simulink model "massdamper"  (R2023a)
settings: Solver=VariableStepAuto  StartTime=0.0  StopTime=10.0  RelTol=1e-3
values from neighbouring files (symbols this model uses):
  k = 1    [RCTF.m]
undefined symbols (not defined in the file or in its folder): b, m
settings Model: Creator=Egypt_Laptop  LastModifiedBy=Egypt_Laptop

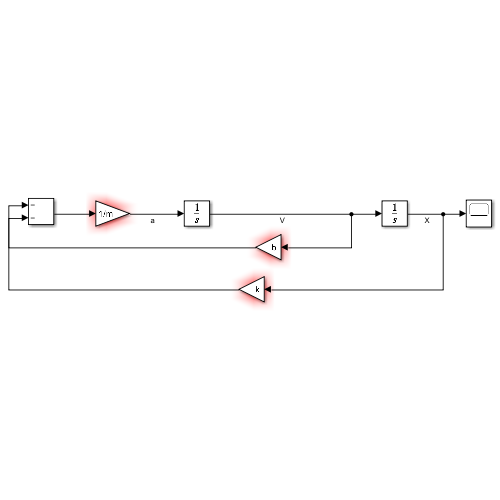
[thumbnail: Simulink's stored preview of the top-level diagram]
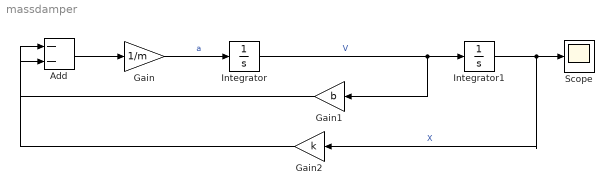
== system massdamper ==
  Add : Sum  Inputs=--
  Gain : Gain  Gain=1/m
  Gain1 : Gain  Gain=b
  Gain2 : Gain  Gain=k
  Integrator : Integrator
  Integrator1 : Integrator
  Scope : Scope
  wires:
  Integrator/1 -> Gain1/1, Integrator1/1  "V"
  Integrator1/1 -> Gain2/1, Scope/1  "X"
  Gain/1 -> Integrator/1  "a"
  Add/1 -> Gain/1
  Gain1/1 -> Add/2
  Gain2/1 -> Add/1
